simulink model "ref_sub_discretefilter_cocoSim_pp"  (R2014b)
settings: Solver=ode45  StartTime=0.0  StopTime=10.0  RelTol=1e-3
settings Model: Creator=arnaud  LastModifiedBy=arnaud
settings DataIOCC: SaveFormat=Structure  SaveOutput=off  SaveTime=off

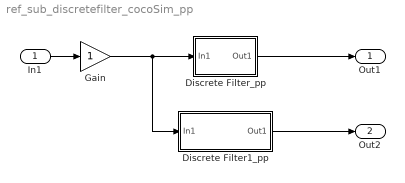
== system ref_sub_discretefilter_cocoSim_pp ==
  In1 : Inport  OutDataTypeStr=double  PortDimensions=1  SampleTime=[1,0]
  Discrete Filter1_pp : Subsystem
  Discrete Filter_pp : Subsystem
  Gain : Gain
  Out1 : Outport  OutDataTypeStr=double  PortDimensions=1  SampleTime=[1,0]
  Out2 : Outport  Port=2  OutDataTypeStr=double  PortDimensions=1  SampleTime=[1,0]
  wires:
  Discrete Filter_pp/1(Out1) -> Out1/1
  Discrete Filter1_pp/1(Out1) -> Out2/1
  In1/1 -> Gain/1
  Gain/1 -> Discrete Filter1_pp/1(In1), Discrete Filter_pp/1(In1)

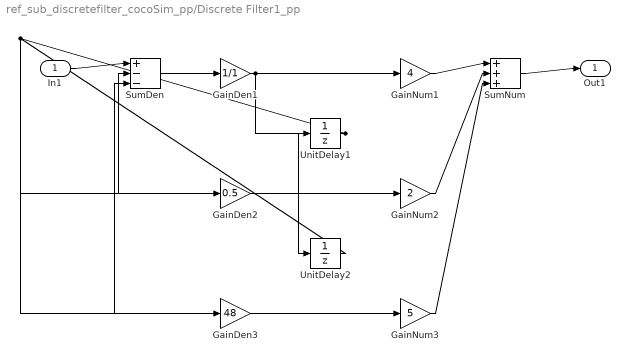
== system ref_sub_discretefilter_cocoSim_pp/Discrete Filter1_pp ==
  In1 : Inport
  GainDen1 : Gain  Gain=1/1  SaturateOnIntegerOverflow=on  OutDataTypeStr=Inherit: Same as input  ParamDataTypeStr=Inherit: Same as input
  GainDen2 : Gain  Gain=0.5  SaturateOnIntegerOverflow=on  OutDataTypeStr=Inherit: Same as input  ParamDataTypeStr=Inherit: Same as input
  GainDen3 : Gain  Gain=48  SaturateOnIntegerOverflow=on  OutDataTypeStr=Inherit: Same as input  ParamDataTypeStr=Inherit: Same as input
  GainNum1 : Gain  Gain=4  SaturateOnIntegerOverflow=on  OutDataTypeStr=Inherit: Same as input  ParamDataTypeStr=Inherit: Same as input
  GainNum2 : Gain  Gain=2  SaturateOnIntegerOverflow=on  OutDataTypeStr=Inherit: Same as input  ParamDataTypeStr=Inherit: Same as input
  GainNum3 : Gain  Gain=5  SaturateOnIntegerOverflow=on  OutDataTypeStr=Inherit: Same as input  ParamDataTypeStr=Inherit: Same as input
  SumDen : Sum  Inputs=+--  SaturateOnIntegerOverflow=on  InputSameDT=on  OutDataTypeStr=Inherit: Same as first input
  SumNum : Sum  Inputs=+++  SaturateOnIntegerOverflow=on  InputSameDT=on  OutDataTypeStr=Inherit: Same as first input
  UnitDelay1 : UnitDelay  InitialCondition=1
  UnitDelay2 : UnitDelay  InitialCondition=0.9
  Out1 : Outport
  wires:
  In1/1 -> SumDen/1
  SumNum/1 -> Out1/1
  SumDen/1 -> GainDen1/1
  GainDen2/1 -> SumDen/2
  GainDen3/1 -> SumDen/3
  GainDen1/1 -> GainNum1/1, UnitDelay1/1
  GainNum1/1 -> SumNum/1
  GainNum2/1 -> SumNum/2
  GainNum3/1 -> SumNum/3
  UnitDelay1/1 -> GainDen2/1, GainNum2/1, UnitDelay2/1
  UnitDelay2/1 -> GainDen3/1, GainNum3/1

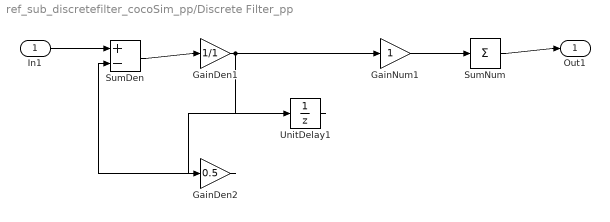
== system ref_sub_discretefilter_cocoSim_pp/Discrete Filter_pp ==
  In1 : Inport
  GainDen1 : Gain  Gain=1/1  SaturateOnIntegerOverflow=on  OutDataTypeStr=Inherit: Same as input  ParamDataTypeStr=Inherit: Same as input
  GainDen2 : Gain  Gain=0.5  SaturateOnIntegerOverflow=on  OutDataTypeStr=Inherit: Same as input  ParamDataTypeStr=Inherit: Same as input
  GainNum1 : Gain  SaturateOnIntegerOverflow=on  OutDataTypeStr=Inherit: Same as input  ParamDataTypeStr=Inherit: Same as input
  SumDen : Sum  Inputs=+-  SaturateOnIntegerOverflow=on  InputSameDT=on  OutDataTypeStr=Inherit: Same as first input
  SumNum : Sum  Inputs=+  SaturateOnIntegerOverflow=on  InputSameDT=on  OutDataTypeStr=Inherit: Same as first input
  UnitDelay1 : UnitDelay
  Out1 : Outport
  wires:
  In1/1 -> SumDen/1
  SumNum/1 -> Out1/1
  SumDen/1 -> GainDen1/1
  GainDen2/1 -> SumDen/2
  GainDen1/1 -> GainNum1/1, UnitDelay1/1
  GainNum1/1 -> SumNum/1
  UnitDelay1/1 -> GainDen2/1
